simulink model "crawldyn1"  (R2019b)
settings: Solver=VariableStepAuto  StartTime=0.0  StopTime=10.0  RelTol=1e-3
libraries: simulink x4
settings Model: Creator=nels-  LastModifiedBy=nels-

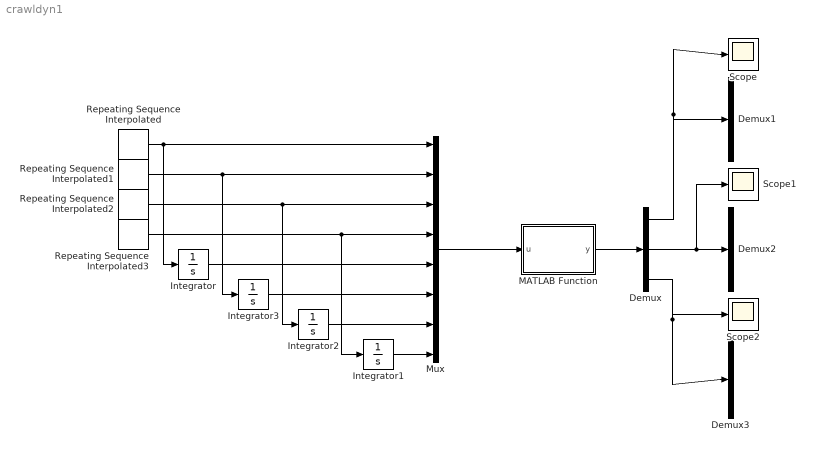
== system crawldyn1 ==
  Demux : Demux  Outputs=3
  Demux1 : Demux
  Demux2 : Demux
  Demux3 : Demux
  Integrator{,1..3} (4 alike) : Integrator
  MATLAB Function : MATLAB Function  TreatAsAtomicUnit=on
  Mux : Mux  Inputs=8
  Repeating Sequence Interpolated : simulink/Sources/Repeating Sequence Interpolated  OutValues=[3 5 7 9 2].'  TimeValues=[0 1 2 3 4].'  LookUpMeth=Interpolation-Use End Values  tsamp=0.01  OutMin=[]  OutMax=[]  OutDataTypeStr=double  OutputDataTypeScalingMode=double  OutDataType=fixdt(0,8)  OutScaling=2^-10
  Repeating Sequence Interpolated1 : simulink/Sources/Repeating Sequence Interpolated  OutValues=[2 9 4].'  TimeValues=[0 1 2].'  LookUpMeth=Interpolation-Use End Values  tsamp=0.01  OutMin=[]  OutMax=[]  OutDataTypeStr=double  OutputDataTypeScalingMode=double  OutDataType=fixdt(0,8)  OutScaling=2^-10
  Repeating Sequence Interpolated2 : simulink/Sources/Repeating Sequence Interpolated  OutValues=[9 5 4 3 7].'  TimeValues=[0 1 2 3 4].'  LookUpMeth=Interpolation-Use End Values  tsamp=0.01  OutMin=[]  OutMax=[]  OutDataTypeStr=double  OutputDataTypeScalingMode=double  OutDataType=fixdt(0,8)  OutScaling=2^-10
  Repeating Sequence Interpolated3 : simulink/Sources/Repeating Sequence Interpolated  OutValues=[9 2 6].'  TimeValues=[0 1 2].'  LookUpMeth=Interpolation-Use End Values  tsamp=0.01  OutMin=[]  OutMax=[]  OutDataTypeStr=double  OutputDataTypeScalingMode=double  OutDataType=fixdt(0,8)  OutScaling=2^-10
  Scope : Scope
  Scope1 : Scope
  Scope2 : Scope
  wires:
  Repeating Sequence Interpolated/1 -> Integrator/1, Mux/1
  Repeating Sequence Interpolated1/1 -> Integrator3/1, Mux/2
  Repeating Sequence Interpolated2/1 -> Integrator2/1, Mux/3
  Repeating Sequence Interpolated3/1 -> Integrator1/1, Mux/4
  Integrator/1 -> Mux/5
  Integrator3/1 -> Mux/6
  Integrator2/1 -> Mux/7
  Integrator1/1 -> Mux/8
  Mux/1 -> MATLAB Function/1(u)
  MATLAB Function/1(y) -> Demux/1
  Demux/1 -> Scope/1, Demux1/1
  Demux/2 -> Scope1/1, Demux2/1
  Demux/3 -> Scope2/1, Demux3/1

== matlab function crawldyn1/MATLAB Function ==
  data: u input; y output
function y=fcn(u)
t1 = deg2rad(u(5));
t2 = deg2rad(u(6));
t3 = deg2rad(u(7));
t4 = deg2rad(u(8));
z=[0; 0; 1];
s1=[0; 0; 55];
s2=[0; 0; 217];
s3=[0; 0; 145];
s4=[0; 0; 30];
sc1=s1/2;
sc2=s2/2;
sc3=s3/2;
sc4=s4/2;


r21=[cos(deg2rad(-90)) -sin(deg2rad(-90)) 0;
     sin(deg2rad(-90))  cos(deg2rad(-90)) 0;
                   0                  0   1];
r22=[1      0        0 ;
     0 cos(t2) -sin(t2);
     0 sin(t2)  cos(t2)];
r2=r21*r22;
r3=[1      0        0 ;
     0 cos(t3) -sin(t3);
     0 sin(t3)  cos(t3)];
r4=[1      0        0 ;
     0 cos(t4) -sin(t4);
     0 sin(t4)  cos(t4)];

 
 
w1=[0; 0; u(1)];
w2=w1+u(2)*r2*z;
w3=w2+u(3)*r3*z;
w4=w3+u(4)*r4*z;

v1=[0; 0; 0];
v2=cross(w2,r2*s2);
v3=v2+cross(w3,r3*s3);
v4=v3+cross(w4,r4*s4);

vc1=[0; 0; 0];
vc2=cross(w2,r2*sc2);
vc3=v2+cross(w3,r3*sc3);
vc4=v3+cross(w4,r4*sc4);

w=[w1; w2; w3; w4];
v=[v1; v2; v3; v4];
vc=[vc1; vc2; vc3; vc4];

y=[w; v; vc]
